simulink model "Worked_Example_9_3"  (R2024b)
settings: Solver=VariableStepAuto  StartTime=0.0  StopTime=1  RelTol=1e-3
settings Model: Creator=GH-X-ST  LastModifiedBy=GH-X-ST

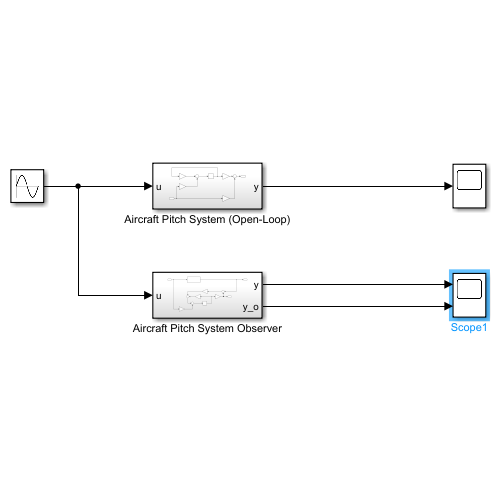
[thumbnail: Simulink's stored preview of the top-level diagram]
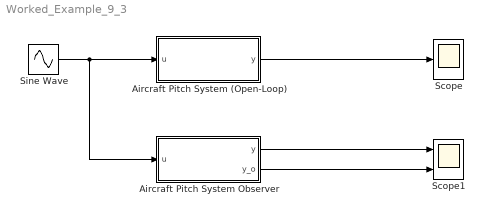
== system Worked_Example_9_3 ==
  Aircraft Pitch System (Open-Loop) : Subsystem
  Aircraft Pitch System Observer : Subsystem
  Scope : Scope
  Scope1 : Scope  NumInputPorts=2
  Sine Wave : Sin  Frequency=3  SampleTime=0
  wires:
  Sine Wave/1 -> Aircraft Pitch System Observer/1(u), Aircraft Pitch System (Open-Loop)/1(u)
  Aircraft Pitch System (Open-Loop)/1(y) -> Scope/1
  Aircraft Pitch System Observer/1(y) -> Scope1/1
  Aircraft Pitch System Observer/2(y_o) -> Scope1/2

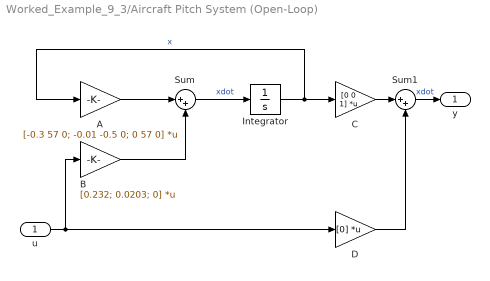
== system Worked_Example_9_3/Aircraft Pitch System (Open-Loop) ==
  u : Inport
  A : Gain  Gain=[-0.3 57 0; -0.01 -0.5 0; 0 57 0]  Multiplication=Matrix(K*u)
  B : Gain  Gain=[0.232; 0.0203; 0]  Multiplication=Matrix(K*u)
  C : Gain  Gain=[0 0 1]  Multiplication=Matrix(K*u)
  D : Gain  Gain=[0]  Multiplication=Matrix(K*u)
  Integrator : Integrator  InitialCondition=[1;1;1]
  Sum : Sum  Inputs=|++
  Sum1 : Sum  Inputs=|++
  y : Outport
  wires:
  u/1 -> D/1, B/1
  A/1 -> Sum/1
  B/1 -> Sum/2
  Sum/1 -> Integrator/1  "xdot"
  Integrator/1 -> C/1, A/1  "x"
  C/1 -> Sum1/1
  Sum1/1 -> y/1  "xdot"
  D/1 -> Sum1/2

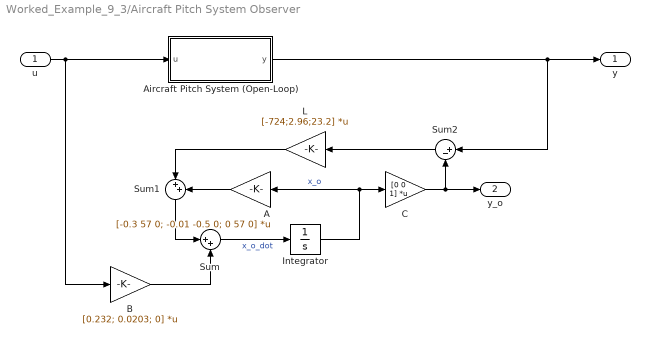
== system Worked_Example_9_3/Aircraft Pitch System Observer ==
  u : Inport
  A : Gain  Gain=[-0.3 57 0; -0.01 -0.5 0; 0 57 0]  Multiplication=Matrix(K*u)
  Aircraft Pitch System (Open-Loop) : Subsystem
  B : Gain  Gain=[0.232; 0.0203; 0]  Multiplication=Matrix(K*u)
  C : Gain  Gain=[0 0 1]  Multiplication=Matrix(K*u)
  Integrator : Integrator  InitialCondition=[0;0;0]
  L : Gain  Gain=[-724;2.96;23.2]  Multiplication=Matrix(K*u)
  Sum : Sum  Inputs=|++
  Sum1 : Sum  Inputs=|++
  Sum2 : Sum  Inputs=|+-
  y : Outport
  y_o : Outport  Port=2
  wires:
  u/1 -> B/1, Aircraft Pitch System (Open-Loop)/1(u)
  Aircraft Pitch System (Open-Loop)/1(y) -> Sum2/1, y/1
  Sum/1 -> Integrator/1  "x_o_dot"
  Integrator/1 -> A/1, C/1  "x_o"
  B/1 -> Sum/2
  Sum1/1 -> Sum/1
  L/1 -> Sum1/1
  A/1 -> Sum1/2
  C/1 -> Sum2/2, y_o/1
  Sum2/1 -> L/1

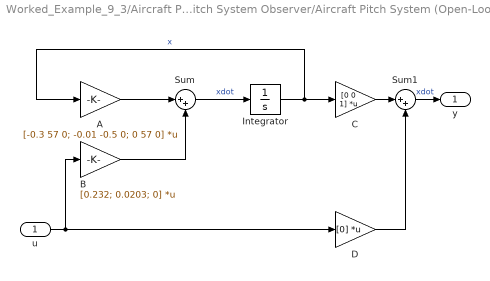
== system Worked_Example_9_3/Aircraft Pitch System Observer/Aircraft Pitch System (Open-Loop) ==
  u : Inport
  A : Gain  Gain=[-0.3 57 0; -0.01 -0.5 0; 0 57 0]  Multiplication=Matrix(K*u)
  B : Gain  Gain=[0.232; 0.0203; 0]  Multiplication=Matrix(K*u)
  C : Gain  Gain=[0 0 1]  Multiplication=Matrix(K*u)
  D : Gain  Gain=[0]  Multiplication=Matrix(K*u)
  Integrator : Integrator  InitialCondition=[1;1;1]
  Sum : Sum  Inputs=|++
  Sum1 : Sum  Inputs=|++
  y : Outport
  wires:
  u/1 -> D/1, B/1
  A/1 -> Sum/1
  B/1 -> Sum/2
  Sum/1 -> Integrator/1  "xdot"
  Integrator/1 -> C/1, A/1  "x"
  C/1 -> Sum1/1
  Sum1/1 -> y/1  "xdot"
  D/1 -> Sum1/2
